simulink model "ejer2_ago31"  (R2016a)
settings: Solver=VariableStepAuto  StartTime=0.0  StopTime=250  RelTol=1e-3
values from neighbouring files (symbols this model uses):
  A = [-B1/M -K/M;1 0]    [ejer2_31Ago.m]    (also in ejer_1_1.m = [0 -1/cap;1/l -r/l]; estabilidad_bibo_marginal.m = 50/((s^2+3)^2*(s^2+5)); linealizacion_multi.m = 2*cos(Theta)./M-(cd*V.^2*L^2*rho)./(2*M))
  B = [1/M ; 0]    [ejer2_31Ago.m]    (also in ejer_1_1.m = [1/cap 0]; estabilidad_bibo_marginal.m = (4*K)/(s^3+3*s^2+2*s+4*K))
  B1 = 0.1    [ejer2_31Ago.m]
  C = 157.58+0.27*s    [ejemplo_pd.m]    (also in ejemplo_pi.m = 0.625+2.375*s+(0.645/s); ejer2_31Ago.m = [0 1]; ejer_1_1.m = [0 r]; segundo_controlador.m = (s-1)/(s+1))
  D = 0    [ejer2_31Ago.m]    (also in ejer_1_1.m)
  K = 0.2    [ejer2_31Ago.m]
  M = 2    [ejer2_31Ago.m]    (also in linealizacion_multi.m = 1; linealizacion_unica.m = 3)
libraries: cstblocks x1
settings Model: Creator=-948  LastModifiedBy=5154922

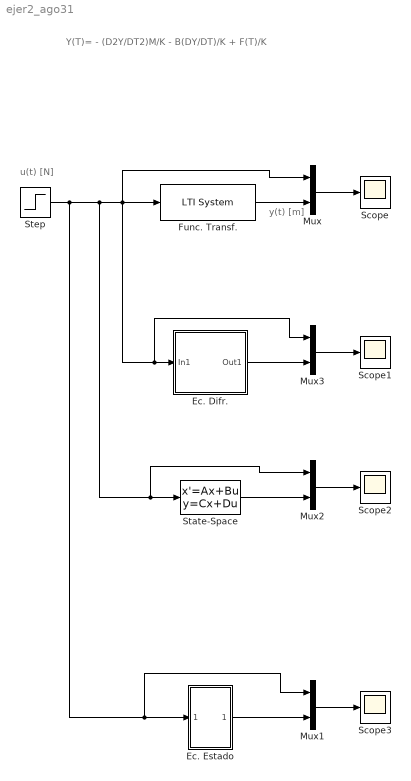
== system ejer2_ago31 ==
  note: Y(T)= - (D2Y/DT2)M/K - B(DY/DT)/K + F(T)/K
  note: y(t) [m]
  note: u(t) [N]
  "Ec. Difr. " : Subsystem
  Ec. Estado : Subsystem
  "Func. Transf. " : cstblocks/LTI System  sys=G  IC=[]
  Mux{,1..3} (4 alike) : Mux  Inputs=2
  Scope{,1..3} (4 alike) : Scope
  State-Space : StateSpace  A=A  B=B  C=C  D=D  X0=0
  Step : Step  SampleTime=0
  wires:
  "Func. Transf. "/1 -> Mux/2
  Mux/1 -> Scope/1
  "Ec. Difr. "/1(Out1) -> Mux3/2
  Step/1 -> Ec. Estado/1(In1), Mux1/1, State-Space/1, Mux2/1, "Ec. Difr. "/1(In1), Mux3/1, Mux/1, "Func. Transf. "/1
  Mux3/1 -> Scope1/1
  State-Space/1 -> Mux2/2
  Mux2/1 -> Scope2/1
  Ec. Estado/1(Out1) -> Mux1/2
  Mux1/1 -> Scope3/1

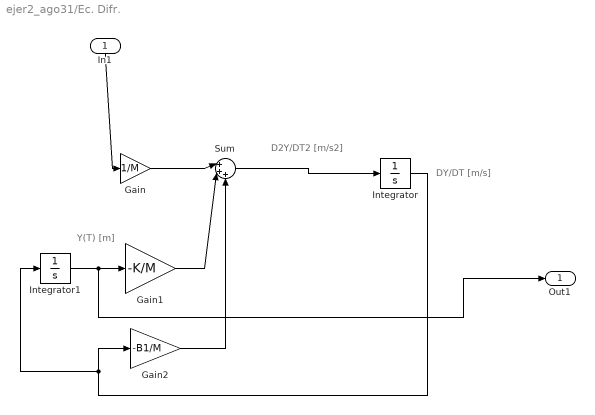
== system ejer2_ago31/Ec. Difr.  ==
  note: Y(T) [m]
  note: DY/DT [m/s]
  note: D2Y/DT2 [m/s2]
  In1 : Inport
  Gain : Gain  Gain=1/M
  Gain1 : Gain  Gain=-K/M
  Gain2 : Gain  Gain=-B1/M
  Integrator : Integrator
  Integrator1 : Integrator
  Sum : Sum  Inputs=|+++
  Out1 : Outport
  wires:
  In1/1 -> Gain/1
  Gain/1 -> Sum/1
  Gain1/1 -> Sum/2
  Integrator1/1 -> Out1/1, Gain1/1
  Sum/1 -> Integrator/1
  Integrator/1 -> Integrator1/1, Gain2/1
  Gain2/1 -> Sum/3

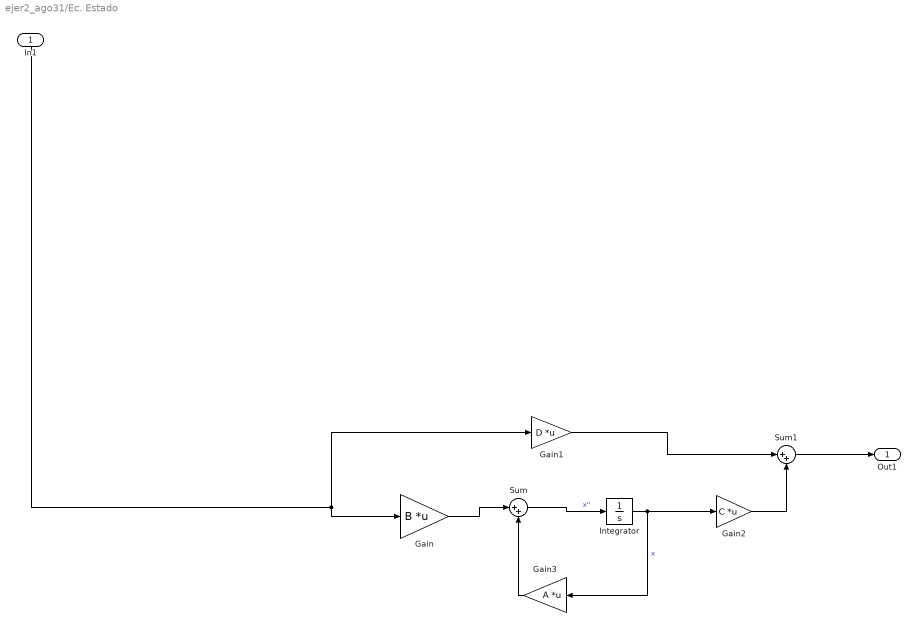
== system ejer2_ago31/Ec. Estado ==
  In1 : Inport
  Gain : Gain  Gain=B  Multiplication=Matrix(K*u)
  Gain1 : Gain  Gain=D  Multiplication=Matrix(K*u)
  Gain2 : Gain  Gain=C  Multiplication=Matrix(K*u)
  Gain3 : Gain  Gain=A  Multiplication=Matrix(K*u)
  Integrator : Integrator
  Sum : Sum  Inputs=|++
  Sum1 : Sum  Inputs=|++
  Out1 : Outport
  wires:
  In1/1 -> Gain1/1, Gain/1
  Sum1/1 -> Out1/1
  Gain/1 -> Sum/1
  Sum/1 -> Integrator/1  "x''"
  Gain2/1 -> Sum1/2
  Integrator/1 -> Gain2/1, Gain3/1  "x"
  Gain3/1 -> Sum/2
  Gain1/1 -> Sum1/1
